simulink model "recibirneopixel"  (R2024b)
settings: Solver=FixedStepDiscrete  StartTime=0.0  StopTime=inf  FixedStep=0.1  RelTol=1e-3  EnableMultiTasking=on
libraries: arduinolib x1, arduinowifilib x1
settings Model: ExtModeTrigDuration=2  Creator=nilsm  LastModifiedBy=nilsm
settings SolverCC: AutoInsertRateTranBlk=on
settings OptimizationCC: EnhancedBackFolding=on  PassReuseOutputArgsAs=Individual arguments  ZeroExternalMemoryAtStartup=off  ZeroInternalMemoryAtStartup=off  MaxStackSize=64  OptimizeBlockOrder=speed  DifferentSizesBufferReuse=on  OptimizationCustomize=off  EfficientTunableParamExpr=on
settings DebuggingCC: ParameterTunabilityLossMsg=error
settings HardwareCC: ProdBitPerPointer=32  ProdBitPerSizeT=32  ProdBitPerPtrDiffT=32  ProdLargestAtomicInteger=Long  ProdLargestAtomicFloat=Double  ProdWordSize=32  ProdHWDeviceType=ARM Compatible->ARM Cortex  UseEmbeddedCoderFeatures=off
settings SFSimCC: MATLABDynamicMemAlloc=off
settings RTWCC: Description=Embedded Coder  SystemTargetFile=ert.tlc  HardwareBoard=ESP32-WROOM(Arduino Compatible)  TLCOptions="-aInlineSetEventsForThisBaseRateFcn=TLC_FALSE -aSuppressMultiTaskScheduler=TLC_FALSE  -aRateBasedStepFcn=0"  TemplateMakefile=ert_default_tmf  CustomInclude=C:/Users/nilsm/Downloads/neopixelcontrol.cpp  Toolchain=ESP32  BuildConfiguration=Faster Runs
settings CodeAppCC: ForceParamTrailComments=on  IgnoreCustomStorageClasses=off  OperatorAnnotations=on  SimulinkDataObjDesc=on  SFDataObjDesc=on  InsertBlockDesc=on
settings ERTTargetCC: SupportContinuousTime=on  SupportNonInlinedSFcns=on  RemoveResetFunc=off  SupportVariableSizeSignals=on  ExtModeTransport=3  ExtModeStaticAlloc=on  ExtModeAutomaticAllocSize=off  ExtModeStaticAllocSize=65536  ExtModeMexFile=ext_xcp  ExtModeIntrfLevel=Level2 - Open  InlinedParameterPlacement=Hierarchical  ConvertIfToSwitch=off  SuppressUnreachableDefaultCases=off

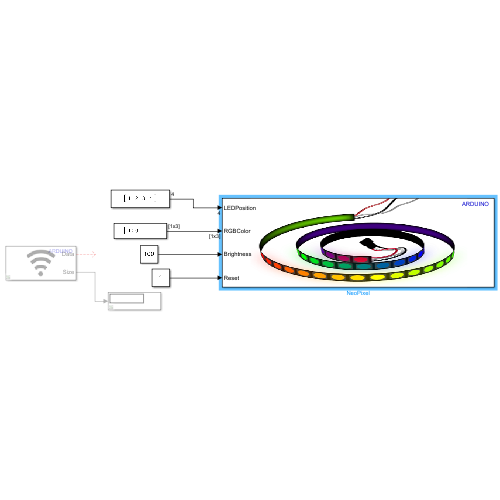
[thumbnail: Simulink's stored preview of the top-level diagram]
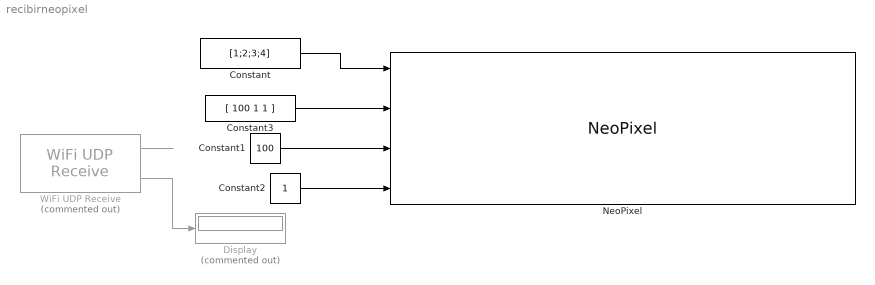
== system recibirneopixel ==
  Constant : Constant  Value=[1;2;3;4]  OutDataTypeStr=uint8
  Constant1 : Constant  Value=100  OutDataTypeStr=uint8
  Constant2 : Constant  OutDataTypeStr=boolean
  Constant3 : Constant  Value=[ 100 1 1 ]  VectorParams1D=off  OutDataTypeStr=uint8
  Display : Display  Commented=on
  NeoPixel : arduinolib/NeoPixel  pin=19  numPixels=15  pixelColor=RGB  pixelFreqType=800KHZ
  WiFi UDP Receive : arduinowifilib/WiFi UDP Receive  Commented=on  localport=8888  DataType=uint8  DataLength=1  SampleTime_=0.1  wifiUDPIndex=0  blockPlatform=ARDUINO  isARMArch=false
  wires:
  Constant2/1 -> NeoPixel/4
  Constant3/1 -> NeoPixel/2
  Constant/1 -> NeoPixel/1
  WiFi UDP Receive/2 -> Display/1
  WiFi UDP Receive/1 -> ?
  Constant1/1 -> NeoPixel/3
